simulink model "MotorXploer"  (R2025b)
settings: Solver=FixedStepAuto  StartTime=0.0  StopTime=30  FixedStep=0.001  RelTol=1e-3
values from neighbouring files (symbols this model uses):
  frequency = frequency(1:min_len)    [openSplitAndEachPlot_Freq.m]    (also in untitled3.m; untitled9.m)
  n = DS.numElements    [spiltefile.m]
undefined symbols (not defined in the file or in its folder): Blocking, LF, Non
libraries: amg_usbconverter_n_connect_lib x3, dspfdesign x1, dspstat3 x1, waijung_addon_module x1
settings Model: Creator=beamk  LastModifiedBy=Asus
settings DebuggingCC: ParameterOverflowMsg=warning  ParameterUnderflowMsg=warning

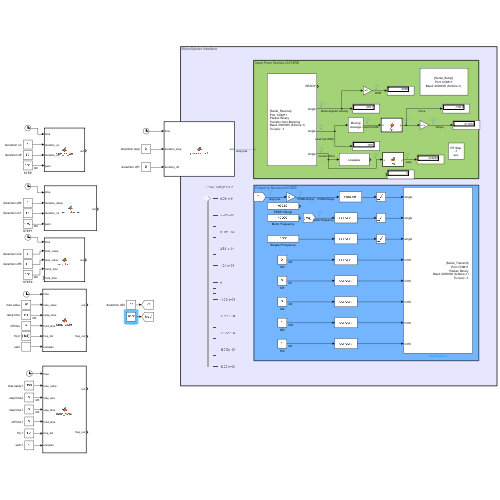
[thumbnail: Simulink's stored preview of the top-level diagram]
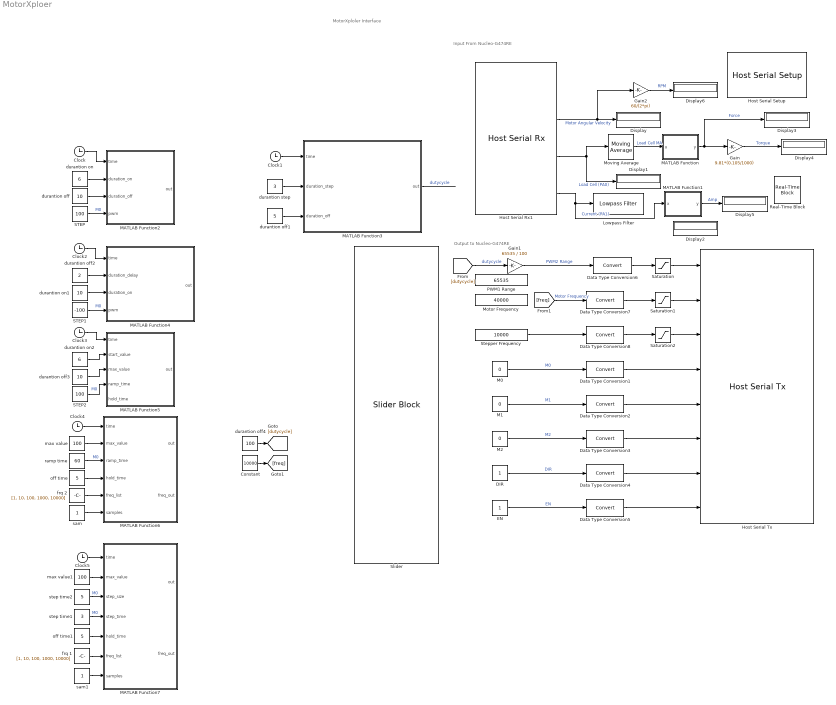
== system MotorXploer ==
  note: Output to Nucleo-G474RE
  note: Input From Nucleo-G474RE
  note: MotorXploler Interface
  Clock{,1..5} (6 alike) : Clock
  Constant : Constant  Value=10000
  DIR : Constant
  Data Type Conversion{1..8} (8 alike) : DataTypeConversion  SaturateOnIntegerOverflow=off  RndMeth=Floor
  Display{,1..6} (7 alike) : Display
  EN : Constant
  Gain : Gain  Gain=9.81*(0.105/1000)
  Gain1 : Gain  Gain=65535 / 100
  Gain2 : Gain  Gain=60/(2*pi)
  Host Serial Rx1 : amg_usbconverter_n_connect_lib/Host Serial Rx  conf=rx  port=<auto>  baudrate=2000000  databits=8  parity=None  stopbit=1  flowcontrol=None  transfer=Non-Blocking  timeout=5  packetmode=Binary  enableinitialvalues=off  initialvalues=[]  binheader='25'  binterminator='4E'  porttype_double=0  porttype_single=3  porttype_int8=0  porttype_uint8=0  porttype_int16=0  porttype_uint16=0  porttype_int32=0  porttype_uint32=0  asciiformat='%f,%f,%d,%d'  rx_asciiterminator="LF (0x0A - \"\\n\")"  tx_asciiterminator="CRLF (0x0D 0x0A - \"\\r\\n\")"  sampletime=0.001  enablecustomportlabel=off  cinputportlabel=0  coutputportlabel=A  portpinstr=0  blockid=HostSerialRx1  inputporttype=[]  inputportwidth=[]  inputportlabel={}  outputporttype=[3 1 1 1]  outputportwidth=[1 1 1 1]  outputportlabel={'READY','single','single','single'}  compat=0  optionstring=[]  autoport='COM11'
  Host Serial Setup : amg_usbconverter_n_connect_lib/Host Serial Setup  conf=setup  port=<auto>  baudrate=2000000  databits=8  parity=None  stopbit=1  flowcontrol=None  transfer=Blocking  timeout=2  packetmode=Binary  initialvalues=[]  binheader='7E 7E'  binterminator='03 03'  porttype_double=0  porttype_single=1  porttype_int8=0  porttype_uint8=0  porttype_int16=0  porttype_uint16=0  porttype_int32=0  porttype_uint32=2  asciiformat='%d %u %x'  rx_asciiterminator="CRLF (0x0D 0x0A - \"\\r\\n\")"  tx_asciiterminator="CRLF (0x0D 0x0A - \"\\r\\n\")"  sampletime=-1  enablecustomportlabel=off  cinputportlabel=0  coutputportlabel=A  portpinstr=0  blockid=HostSerialSetup  inputporttype=[]  inputportwidth=[]  inputportlabel={}  outputporttype=[]  outputportwidth=[]  outputportlabel={}  compat=0  optionstring=[]  autoport='COM11'
  Host Serial Tx : amg_usbconverter_n_connect_lib/Host Serial Tx  conf=tx  port=<auto>  baudrate=2000000  databits=8  parity=None  stopbit=1  flowcontrol=None  transfer=Blocking  timeout=2  packetmode=Binary  initialvalues=[]  binheader='25'  binterminator='4E'  porttype_double=0  porttype_single=3  porttype_int8=0  porttype_uint8=0  porttype_int16=5  porttype_uint16=0  porttype_int32=0  porttype_uint32=0  asciiformat='%d,%f'  rx_asciiterminator="CRLF (0x0D 0x0A - \"\\r\\n\")"  tx_asciiterminator="CRLF (0x0D 0x0A - \"\\r\\n\")"  sampletime=0.001  enablecustomportlabel=off  cinputportlabel=0  coutputportlabel=A  portpinstr=0  blockid=HostSerialTx  inputporttype=[1 1 1 4 4 4 4 4]  inputportwidth=[1 1 1 1 1 1 1 1]  inputportlabel={'single','single','single','int16','int16','int16','int16','int16'}  outputporttype=[]  outputportwidth=[]  outputportlabel={}  compat=0  optionstring=[]  autoport='COM11'
      settings: SourceProductName=aMG USB Converter N
  Lowpass Filter : dspfdesign/Lowpass Filter  FilterType=FIR  DesignForMinimumOrder=on  FilterOrder=50  PassbandFrequency=0.02  StopbandFrequency=0.04  PassbandRipple=0.1  StopbandAttenuation=80  SampleRateMode=Use normalized frequency (0 to 1)  SampleRate=44100  SimulateUsing=Interpreted execution  roundingMode=Floor  coeffsDataTypeStr=fixdt(1,16)
  M0 : Constant  Value=0
  M1 : Constant  Value=0
  M2 : Constant  Value=0
  MATLAB Function : MATLAB Function  TreatAsAtomicUnit=on
  MATLAB Function1 : MATLAB Function  TreatAsAtomicUnit=on
  MATLAB Function2 : MATLAB Function  TreatAsAtomicUnit=on
  MATLAB Function3 : MATLAB Function  TreatAsAtomicUnit=on
  MATLAB Function4 : MATLAB Function  TreatAsAtomicUnit=on
  MATLAB Function5 : MATLAB Function  TreatAsAtomicUnit=on
  MATLAB Function6 : MATLAB Function  TreatAsAtomicUnit=on
  MATLAB Function7 : MATLAB Function  TreatAsAtomicUnit=on
  Motor Frequency : Constant  Value=40000  OutDataTypeStr=single
  Moving Average : dspstat3/Moving Average  Method=Sliding window  ForgettingFactorPort=off  SpecifyWindowLength=on  WindowLength=1000  OverlapLength=999  AllowArbitraryInputLength=off  ForgettingFactor=0.9  SimulateUsing=Interpreted execution
  PWM1 Range : Constant  Value=65535  VectorParams1D=off  OutDataTypeStr=single
  Real-Time Block : waijung_addon_module/Real-Time Block  Priority=0  setting=Default  sampletime=-1
      settings: SourceProductName=Misc
  STEP : Constant  Value=100
  STEP1 : Constant  Value=-100
  STEP2 : Constant  Value=100
  Saturation : Saturate  UpperLimit=65535  LowerLimit=-65535
  Saturation1 : Saturate  UpperLimit=20000  LowerLimit=0
  Saturation2 : Saturate  UpperLimit=inf  LowerLimit=0
  Slider : SliderBlock  ScaleMin=-65535  ScaleMax=65535
  Stepper Frequency : Constant  Value=10000  OutDataTypeStr=single
  durantion off : Constant  Value=10
  durantion off1 : Constant  Value=5
  durantion off2 : Constant  Value=2
  durantion off3 : Constant  Value=10
  durantion off4 : Constant  Value=100
  durantion on : Constant  Value=6
  durantion on1 : Constant  Value=10
  durantion on2 : Constant  Value=6
  durantion step : Constant  Value=3
  frq 1 : Constant  Value=[1, 10, 100, 1000, 10000]
  frq 2 : Constant  Value=[1, 10, 100, 1000, 10000]
  max value : Constant  Value=100
  max value1 : Constant  Value=100
  off time : Constant  Value=5
  off time1 : Constant  Value=5
  ramp time : Constant  Value=60
  sam : Constant
  sam1 : Constant
  step time1 : Constant  Value=3
  step time2 : Constant  Value=5
  wires:
  Host Serial Rx1/2 -> Gain2/1, Display/1  "Motor Angular Velocity"
  Host Serial Rx1/3 -> Moving Average/1, Display1/1  "Load Cell (PA0)"
  M0/1 -> Data Type Conversion1/1  "M0"
  EN/1 -> Data Type Conversion5/1  "EN"
  DIR/1 -> Data Type Conversion4/1  "DIR"
  M1/1 -> Data Type Conversion2/1  "M1"
  M2/1 -> Data Type Conversion3/1  "M2"
  Stepper Frequency/1 -> Data Type Conversion8/1
  Data Type Conversion1/1 -> Host Serial Tx/4
  Data Type Conversion2/1 -> Host Serial Tx/5
  Data Type Conversion3/1 -> Host Serial Tx/6
  Data Type Conversion4/1 -> Host Serial Tx/7
  Data Type Conversion5/1 -> Host Serial Tx/8
  Saturation/1 -> Host Serial Tx/1
  Data Type Conversion7/1 -> Saturation1/1
  Data Type Conversion8/1 -> Saturation2/1
  Saturation1/1 -> Host Serial Tx/2
  Saturation2/1 -> Host Serial Tx/3
  MATLAB Function/1(y) -> Gain/1, Display3/1  "Force"
  Moving Average/1 -> MATLAB Function/1(u)  "Load Cell MA"
  Gain/1 -> Display4/1  "Torque"
  MATLAB Function1/1(y) -> Display5/1  "Amp"
  Gain2/1 -> Display6/1  "RPM"
  STEP/1 -> MATLAB Function2/4(pwm)  "M0"
  durantion on/1 -> MATLAB Function2/2(duration_on)
  durantion off/1 -> MATLAB Function2/3(duration_off)
  Clock/1 -> MATLAB Function2/1(time)
  Clock1/1 -> MATLAB Function3/1(time)
  durantion step/1 -> MATLAB Function3/2(duration_step)
  durantion off1/1 -> MATLAB Function3/3(duration_off)
  Data Type Conversion6/1 -> Saturation/1
  durantion off2/1 -> MATLAB Function4/2(duration_delay)
  Clock2/1 -> MATLAB Function4/1(time)
  STEP1/1 -> MATLAB Function4/4(pwm)  "M0"
  durantion on1/1 -> MATLAB Function4/3(duration_on)
  Host Serial Rx1/4 -> Lowpass Filter/1, MATLAB Function1/1(x)  "Current (PA1)"
  Gain1/1 -> Data Type Conversion6/1  "PWM2 Range"
  durantion off3/1 -> MATLAB Function5/3(max_value)
  Clock3/1 -> MATLAB Function5/1(time)
  STEP2/1 -> MATLAB Function5/4(ramp_time)  "M0"
  durantion on2/1 -> MATLAB Function5/2(start_value)
  frq 2/1 -> MATLAB Function6/5(freq_list)
  max value/1 -> MATLAB Function6/2(max_value)
  ramp time/1 -> MATLAB Function6/3(ramp_time)  "M0"
  Clock4/1 -> MATLAB Function6/1(time)
  MATLAB Function3/1(out) -> ?  "dutycycle"
  off time/1 -> MATLAB Function6/4(hold_time)
  sam/1 -> MATLAB Function6/6(samples)
  [dutycycle] -> Gain1/1  "dutycycle"
  [freq] -> Data Type Conversion7/1  "Motor Frequency"
  Clock5/1 -> MATLAB Function7/1(time)
  step time1/1 -> MATLAB Function7/4(step_time)  "M0"
  off time1/1 -> MATLAB Function7/5(hold_time)
  max value1/1 -> MATLAB Function7/2(max_value)
  frq 1/1 -> MATLAB Function7/6(freq_list)
  sam1/1 -> MATLAB Function7/7(samples)
  step time2/1 -> MATLAB Function7/3(step_size)  "M0"
  durantion off4/1 -> [dutycycle]
  Constant/1 -> [freq]

== matlab function MotorXploer/MATLAB Function1 ==
  data: x input; y output
function y = fcn(x)

y = (x - 2112.2) / 29.469 ;

== matlab function MotorXploer/MATLAB Function ==
  data: u input; y output
function y = fcn(u)
y = (0.2788*u + 113.58) - 495 -56;

== matlab function MotorXploer/MATLAB Function2 ==
  data: time input; out output; duration_on input; duration_off input; pwm input
function out= pwm_on_off(time, duration_on, duration_off, pwm)
% t = current simulation time
% duration_on = เวลาที่ต้องการให้จ่าย pwm
% duration_off = เวลาที่ต้องการให้ปิด (0)
% pwm = ค่าที่ต้องการจ่ายเมื่ออยู่ในช่วง on
        cycle = duration_on + duration_off;
    
        % ป้องกันค่า cycle = 0
        if cycle <= 0
            out = 0;
            return;
        end
    
        % หาว่าเวลาปัจจุบันอยู่ตำแหน่งใดในรอบ
        t_mod = mod(time, cycle);
    
        % ช่วง on
        if t_mod < duration_on
            out = pwm;
        else
            out = 0;
        end
    end

== matlab function MotorXploer/MATLAB Function3 ==
  data: time input; out output; duration_step input; duration_off input
function out  = pwm_on_off(time, duration_step, duration_off)
% t = current simulation time
% duration_on = เวลาที่ต้องการให้จ่าย pwm
% duration_off = เวลาที่ต้องการให้ปิด (0)
% pwm = ค่าที่ต้องการจ่ายเมื่ออยู่ในช่วง on
        duration_on = (duration_step * 20);
        cycle = duration_on + duration_off;
    
        % ป้องกันค่า cycle = 0
        if cycle <= 0
            out = 0;
            return;
        end
    
        % หาว่าเวลาปัจจุบันอยู่ตำแหน่งใดในรอบ
        t_mod = mod(time, cycle);
    
        % ช่วง on
        if t_mod < duration_on
            out = (floor(t_mod / duration_step) + 1) * 5;
        else
            out = 0;
        end
    end

== matlab function MotorXploer/MATLAB Function4 ==
  data: time input; duration_delay input; out output; duration_on input; pwm input
function out = pwm_delay_on(time, duration_delay, duration_on, pwm)
        out = 0;
        if time >= duration_delay + duration_on 
            return;
        end
        if time >= duration_delay
            out = pwm;
            return;
        end   
end

== matlab function MotorXploer/MATLAB Function5 ==
  data: time input; out output; start_value input; max_value input; ramp_time input; hold_time input
function out = ramp_hold(time, start_value, max_value, ramp_time, hold_time)
    % ตั้งค่า default
    out = start_value;

    % ป้องกัน ramp_time <= 0
    if ramp_time <= 0
        out = max_value;
        return;
    end

    % ช่วงเร่งจาก start → max
    if time < ramp_time
        rate = (max_value - start_value) / ramp_time;
        out = start_value + rate * time;
        return;
    end

    % ช่วงคงที่บน
    if time < ramp_time + hold_time
        out = max_value;
        return;
    end

    % หลังจาก hold_time จบ ลงท้ายด้วยคงค่าสูงสุด
    out = max_value;
end

== matlab function MotorXploer/MATLAB Function6 ==
  data: time input; max_value input; ramp_time input; hold_time input; out output; freq_list input; freq_out output; samples input
function [out, freq_out] = ramp_cycle(time, max_value, ramp_time, hold_time, freq_list, samples)
    % output default
    out = 0;
    freq_out = 0;

    n = length(freq_list);
    if n == 0
        return;
    end

    % เวลาของหนึ่ง cycle
    one_cycle = hold_time + ramp_time;

    if one_cycle <= 0
        return;
    end

    % เวลา 3 cycle
    three_cycles = samples * one_cycle;

    % หา index ของ freq_out ปัจจุบัน
    idx = floor(time / three_cycles) + 1;

    if idx > n
        idx = n;
    end

    freq_out = freq_list(idx);

    % เวลาใน cycle ปัจจุบัน (ไม่สน cycle อื่น)
    t_mod = mod(time, one_cycle);

    % โซน 1: hold ที่ 0
    if t_mod < hold_time
        out = 0;
        return;
    end

    % โซน 2: ramp จาก 0 → max_value
    if t_mod < hold_time + ramp_time
        t_ramp = t_mod - hold_time;
        rate = max_value / ramp_time;
        out = rate * t_ramp;
        return;
    end

    % โซน 3: hold max
    out = 0;
end

== matlab function MotorXploer/MATLAB Function7 ==
  data: time input; max_value input; step_size input; step_time input; hold_time input; out output; freq_list input; freq_out output; samples input
function [out, freq_out] = ramp_cycle(time, max_value, step_size, step_time, hold_time, freq_list, samples)
    % output default
    out = 0;
    freq_out = 0;

    n = length(freq_list);
    if n == 0
        return;
    end

    % เวลาของหนึ่ง cycle
    one_cycle = hold_time + ((max_value / step_size) * step_time);

    if one_cycle <= 0
        return;
    end

    % เวลา 3 cycle
    three_cycles = samples * one_cycle;

    % หา index ของ freq_out ปัจจุบัน
    idx = floor(time / three_cycles) + 1;

    if idx > n
        idx = n;
    end

    freq_out = freq_list(idx);

    % เวลาใน cycle ปัจจุบัน (ไม่สน cycle อื่น)
    t_mod = mod(time, one_cycle);

    % โซน 1: hold ที่ 0
    if t_mod < hold_time
        out = 0;
        return;
    end

    % โซน 2: ramp จาก 0 → max_value
    if t_mod < hold_time + ((max_value / step_size) * step_time)
        t_step = t_mod - hold_time;
        rate = 1 + floor(t_step / step_time);
        out = rate * step_size;
        return;
    end

    % โซน 3: hold max
    out = max_value;
end
